simulink model "RLC"  (R2023a)
settings: Solver=VariableStepAuto  StartTime=0.0  StopTime=1  RelTol=1e-8
values from neighbouring files (symbols this model uses):
  C = 1    [constants.m]
  L = 2    [constants.m]
  R = 1    [constants.m]
settings Model: Creator=Researcher  LastModifiedBy=Researcher

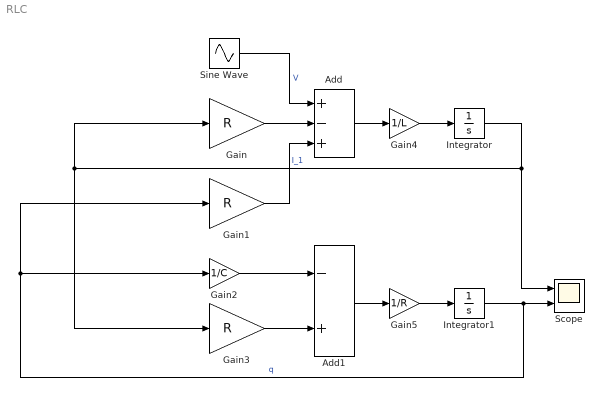
== system RLC ==
  Add : Sum  Inputs=+-+
  Add1 : Sum  Inputs=-+
  Gain : Gain  Gain=R
  Gain1 : Gain  Gain=R
  Gain2 : Gain  Gain=1/C
  Gain3 : Gain  Gain=R
  Gain4 : Gain  Gain=1/L
  Gain5 : Gain  Gain=1/R
  Integrator : Integrator
  Integrator1 : Integrator
  Scope : Scope  NumInputPorts=2
  Sine Wave : Sin  Amplitude=220  Frequency=100*pi  SampleTime=0
  wires:
  Integrator/1 -> Gain3/1, Gain/1, Scope/1  "I_1"
  Gain/1 -> Add/2
  Gain1/1 -> Add/3
  Sine Wave/1 -> Add/1  "V"
  Integrator1/1 -> Gain2/1, Gain1/1, Scope/2  "q"
  Gain2/1 -> Add1/1
  Gain3/1 -> Add1/2
  Add/1 -> Gain4/1
  Add1/1 -> Gain5/1
  Gain5/1 -> Integrator1/1
  Gain4/1 -> Integrator/1
